simulink model "Obs_L"  (R2025b)
settings: Solver=VariableStepAuto  StartTime=0.0  StopTime=500  RelTol=1e-3
values from neighbouring files (symbols this model uses):
  AL = A-L*C    [fase1.m]
  BL = [Bu L]    [fase1.m]
  C = [1, 0, 0]    [fase1.m]
  CL = eye(size(A))    [fase1.m]
  DL = zeros(size(A,1),2)    [fase1.m]
  yeq = xeq(1,:)    [fase1.m]
undefined symbols (not defined in the file or in its folder): ueq, xeq
settings Model: Creator=Rika  LastModifiedBy=Rika

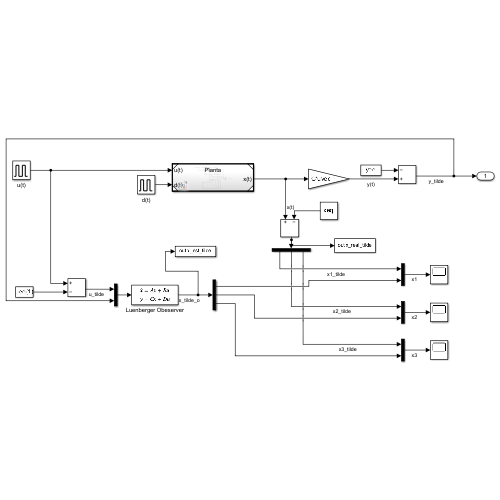
[thumbnail: Simulink's stored preview of the top-level diagram]
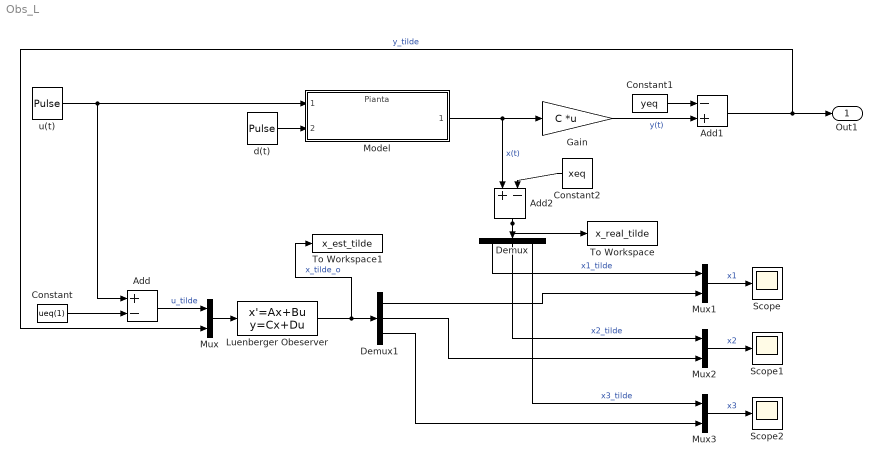
== system Obs_L ==
  Add : Sum  Inputs=+-
  Add1 : Sum  Inputs=-+
  Add2 : Sum  Inputs=+-
  Constant : Constant  Value=ueq(1)
  Constant1 : Constant  Value=yeq
  Constant2 : Constant  Value=xeq
  Demux : Demux  Outputs=3
  Demux1 : Demux  Outputs=3
  Gain : Gain  Gain=C  Multiplication=Matrix(K*u) (u vector)
  Luenberger Obeserver : StateSpace  A=AL  B=BL  C=CL  D=DL  InitialCondition=0
  Model : ModelReference  ModelNameDialog=Pianta.slx  SimulationMode=Normal  ModelReferenceVersion=1.16
  Mux{,1..3} (4 alike) : Mux  Inputs=2
  Scope : Scope
      settings: ActiveDisplayYMinimum=-137.10991668616327  ActiveDisplayYMaximum=515.3842187499622
  Scope1 : Scope
      settings: ActiveDisplayYMinimum=-0.086960897476082669  ActiveDisplayYMaximum=0.038438023602776428
  Scope2 : Scope
      settings: ActiveDisplayYMinimum=-122.27598794510493  ActiveDisplayYMaximum=87.090569847303414  DataLoggingVariableName=ScopeData2
  To Workspace : ToWorkspace  VariableName=x_real_tilde  SampleTime=-1
  To Workspace1 : ToWorkspace  VariableName=x_est_tilde  SampleTime=-1
  d(t) : DiscretePulseGenerator  PulseType=Time based  Amplitude=10  Period=1000  PulseWidth=3  PhaseDelay=10
  u(t) : DiscretePulseGenerator  PulseType=Time based  Amplitude=15  Period=1000  PulseWidth=0.5  PhaseDelay=10
  Out1 : Outport
  wires:
  Mux/1 -> Luenberger Obeserver/1
  Add/1 -> Mux/1  "u_tilde"
  Add1/1 -> Mux/2, Out1/1  "y_tilde"
  Gain/1 -> Add1/2  "y(t)"
  d(t)/1 -> Model/2
  Constant1/1 -> Add1/1
  Model/1 -> Add2/1, Gain/1  "x(t)"
  Constant2/1 -> Add2/2
  Add2/1 -> To Workspace/1, Demux/1
  Luenberger Obeserver/1 -> To Workspace1/1, Demux1/1  "x_tilde_o"
  Mux1/1 -> Scope/1  "x1"
  Demux/1 -> Mux1/1  "x1_tilde"
  Demux1/1 -> Mux1/2
  Mux2/1 -> Scope1/1  "x2"
  Mux3/1 -> Scope2/1  "x3"
  Demux/2 -> Mux2/1  "x2_tilde"
  Demux1/2 -> Mux2/2
  Demux1/3 -> Mux3/2
  Demux/3 -> Mux3/1  "x3_tilde"
  u(t)/1 -> Add/1, Model/1
  Constant/1 -> Add/2
